simulink model "PQ_VSC_complete_v1"  (R2013b)
settings: Solver=ode45  StartTime=0.0  StopTime=2  MaxStep=0.001  RelTol=1e-3
values from neighbouring files (symbols this model uses):
  Ki = 100    [data_PQsharing.m]
  Ki_PLL = (2*pi*200)^2    (= 1579136.70417)    [data_PQsharing.m]
  Ki_pq = 20    [data_PQsharing.m]
  Kp = 50    [data_PQsharing.m]
  Kp_PLL = sqrt(Ki_PLL)*0.2    [data_PQsharing.m]
  Kp_pq = 0.1    [data_PQsharing.m]
  L = L1    (= 0.04)    [data_PQsharing.m]
  R = 1    [data_PQsharing.m]
  w0 = 377    [data_PQsharing.m]
settings Model: Creator=linglingfan  LastModifiedBy=linglingfan

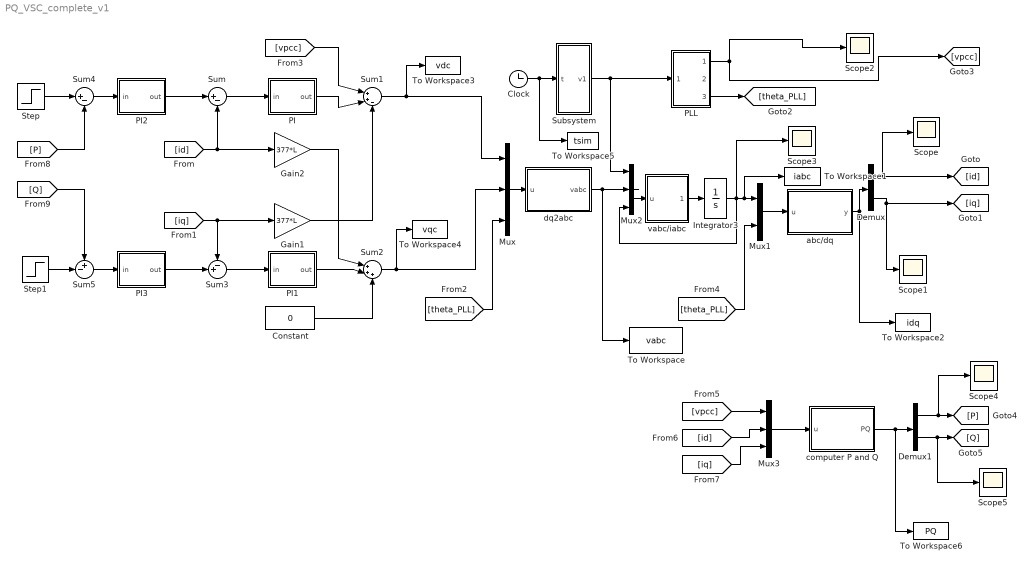
== system PQ_VSC_complete_v1 ==
  Clock : Clock
  Constant : Constant  Value=0
  Demux : Demux  Outputs=2
  Demux1 : Demux  Outputs=2
  Gain1 : Gain  Gain=377*L
  Gain2 : Gain  Gain=377*L
  Integrator3 : Integrator  InitialCondition=zeros(3,1)
  Mux : Mux  Inputs=3
  Mux1 : Mux  Inputs=2
  Mux2 : Mux  Inputs=3
  Mux3 : Mux  Inputs=3
  PI : Subsystem
  PI1 : Subsystem
  PI2 : Subsystem
  PI3 : Subsystem
  PLL : Subsystem
  Scope{,1..5} (6 alike) : Scope
      Scope2 settings: SaveName=ScopeData2
      Scope3 settings: SaveName=ScopeData3
      Scope4 settings: YMin=-6  YMax=7  SaveName=ScopeData4
      Scope5 settings: SaveName=ScopeData5
  Step : Step  Time=0.25  After=0.1  SampleTime=0
  Step1 : Step  After=0.1  SampleTime=0
  Subsystem : Subsystem
  Sum : Sum  Inputs=|+-
  Sum1 : Sum  Inputs=|++-
  Sum2 : Sum  Inputs=|+++
  Sum3 : Sum  Inputs=-+|
  Sum4 : Sum  Inputs=|+-
  Sum5 : Sum  Inputs=+-|
  To Workspace : ToWorkspace  VariableName=vabc  SampleTime=-1
  To Workspace1 : ToWorkspace  VariableName=iabc  SampleTime=-1
  To Workspace2 : ToWorkspace  VariableName=idq  SampleTime=-1
  To Workspace3 : ToWorkspace  VariableName=vdc  SampleTime=-1
  To Workspace4 : ToWorkspace  VariableName=vqc  SampleTime=-1
  To Workspace5 : ToWorkspace  VariableName=tsim  SampleTime=-1
  To Workspace6 : ToWorkspace  VariableName=PQ  SampleTime=-1
  abc/dq : MATLAB Function  TreatAsAtomicUnit=on
  computer P and Q : MATLAB Function  TreatAsAtomicUnit=on
  dq2abc : MATLAB Function  TreatAsAtomicUnit=on
  vabc/iabc : MATLAB Function  TreatAsAtomicUnit=on
  wires:
  Sum/1 -> PI/1(in)
  Mux/1 -> dq2abc/1(u)
  vabc/iabc/1(d_iabc) -> Integrator3/1
  Mux1/1 -> abc/dq/1(u)
  Demux/1 -> Scope/1, [id]
  Demux/2 -> Scope1/1, [iq]
  [id] -> Gain2/1, Sum/2
  [iq] -> Sum3/1, Gain1/1
  Gain2/1 -> Sum2/1
  PI1/1(out) -> Sum2/2
  Constant/1 -> Sum2/3
  [vpcc] -> Sum1/1
  PI/1(out) -> Sum1/2
  Gain1/1 -> Sum1/3
  Sum3/1 -> PI1/1(in)
  PI3/1(out) -> Sum3/2
  PI2/1(out) -> Sum/1
  Sum2/1 -> To Workspace4/1, Mux/2
  Sum1/1 -> To Workspace3/1, Mux/1
  Clock/1 -> To Workspace5/1, Subsystem/1(t)
  Mux2/1 -> vabc/iabc/1(u)
  Subsystem/1(v1) -> PLL/1(abc), Mux2/1
  Integrator3/1 -> Scope3/1, To Workspace1/1, Mux1/1, Mux2/3
  PLL/3(ang) -> [theta_PLL]
  [theta_PLL] -> Mux/3
  dq2abc/1(vabc) -> To Workspace/1, Mux2/2
  PLL/1(mag) -> Scope2/1, [vpcc]
  [theta_PLL] -> Mux1/2
  abc/dq/1(y) -> Demux/1, To Workspace2/1
  [vpcc] -> Mux3/1
  [id] -> Mux3/2
  [iq] -> Mux3/3
  Mux3/1 -> computer P and Q/1(u)
  computer P and Q/1(PQ) -> To Workspace6/1, Demux1/1
  Demux1/1 -> Scope4/1, [P]
  Demux1/2 -> Scope5/1, [Q]
  Sum4/1 -> PI2/1(in)
  Sum5/1 -> PI3/1(in)
  [P] -> Sum4/2
  [Q] -> Sum5/1
  Step/1 -> Sum4/1
  Step1/1 -> Sum5/2

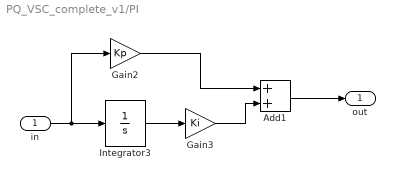
== system PQ_VSC_complete_v1/PI ==
  in : Inport
  Add1 : Sum
  Gain2 : Gain  Gain=Kp
  Gain3 : Gain  Gain=Ki
  Integrator3 : Integrator
  out : Outport
  wires:
  Add1/1 -> out/1
  in/1 -> Gain2/1, Integrator3/1
  Gain3/1 -> Add1/2
  Gain2/1 -> Add1/1
  Integrator3/1 -> Gain3/1

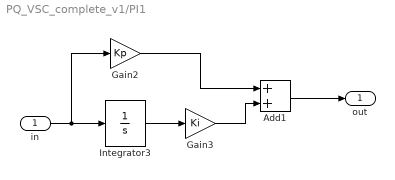
== system PQ_VSC_complete_v1/PI1 ==
  in : Inport
  Add1 : Sum
  Gain2 : Gain  Gain=Kp
  Gain3 : Gain  Gain=Ki
  Integrator3 : Integrator
  out : Outport
  wires:
  Add1/1 -> out/1
  in/1 -> Gain2/1, Integrator3/1
  Gain3/1 -> Add1/2
  Gain2/1 -> Add1/1
  Integrator3/1 -> Gain3/1

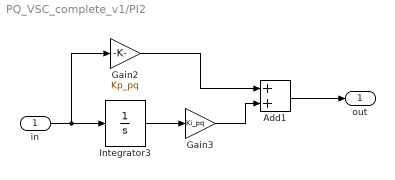
== system PQ_VSC_complete_v1/PI2 ==
  in : Inport
  Add1 : Sum
  Gain2 : Gain  Gain=Kp_pq
  Gain3 : Gain  Gain=Ki_pq
  Integrator3 : Integrator
  out : Outport
  wires:
  Add1/1 -> out/1
  in/1 -> Gain2/1, Integrator3/1
  Gain3/1 -> Add1/2
  Gain2/1 -> Add1/1
  Integrator3/1 -> Gain3/1

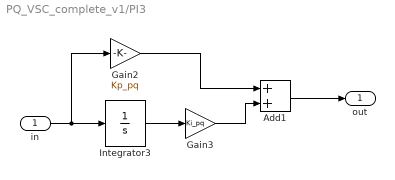
== system PQ_VSC_complete_v1/PI3 ==
  in : Inport
  Add1 : Sum
  Gain2 : Gain  Gain=Kp_pq
  Gain3 : Gain  Gain=Ki_pq
  Integrator3 : Integrator
  out : Outport
  wires:
  Add1/1 -> out/1
  in/1 -> Gain2/1, Integrator3/1
  Gain3/1 -> Add1/2
  Gain2/1 -> Add1/1
  Integrator3/1 -> Gain3/1

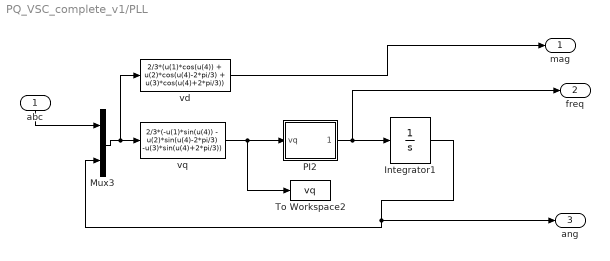
== system PQ_VSC_complete_v1/PLL ==
  abc : Inport
  Integrator1 : Integrator
  Mux3 : Mux  Inputs=2
  PI2 : Subsystem
  To Workspace2 : ToWorkspace  VariableName=vq  SampleTime=-1
  vd : Fcn  Expr=2/3*(u(1)*cos(u(4)) + u(2)*cos(u(4)-2*pi/3) + u(3)*cos(u(4)+2*pi/3))
  vq : Fcn  Expr=2/3*(-u(1)*sin(u(4)) - u(2)*sin(u(4)-2*pi/3) -u(3)*sin(u(4)+2*pi/3))
  mag : Outport
  freq : Outport  Port=2
  ang : Outport  Port=3
  wires:
  Mux3/1 -> vd/1, vq/1
  PI2/1(omega) -> freq/1, Integrator1/1
  abc/1 -> Mux3/1
  vq/1 -> To Workspace2/1, PI2/1(vq)
  vd/1 -> mag/1
  Integrator1/1 -> ang/1, Mux3/2

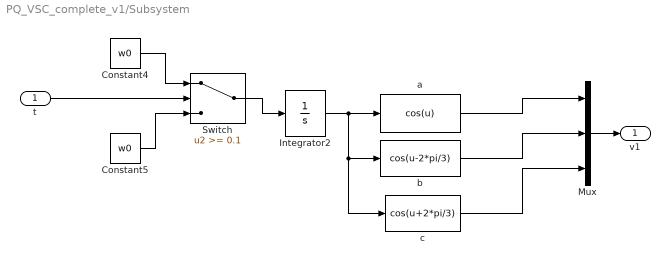
== system PQ_VSC_complete_v1/Subsystem ==
  t : Inport
  Constant4 : Constant  Value=w0
  Constant5 : Constant  Value=w0
  Integrator2 : Integrator
  Mux : Mux  Inputs=3
  Switch : Switch  Threshold=0.1
  a : Fcn  Expr=cos(u)
  b : Fcn  Expr=cos(u-2*pi/3)
  c : Fcn  Expr=cos(u+2*pi/3)
  v1 : Outport
  wires:
  a/1 -> Mux/1
  c/1 -> Mux/3
  Integrator2/1 -> c/1, b/1, a/1
  b/1 -> Mux/2
  t/1 -> Switch/2
  Constant4/1 -> Switch/1
  Switch/1 -> Integrator2/1
  Constant5/1 -> Switch/3
  Mux/1 -> v1/1

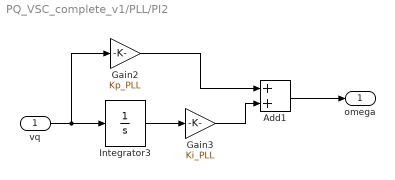
== system PQ_VSC_complete_v1/PLL/PI2 ==
  vq : Inport
  Add1 : Sum
  Gain2 : Gain  Gain=Kp_PLL
  Gain3 : Gain  Gain=Ki_PLL
  Integrator3 : Integrator
  omega : Outport
  wires:
  Add1/1 -> omega/1
  vq/1 -> Gain2/1, Integrator3/1
  Gain3/1 -> Add1/2
  Gain2/1 -> Add1/1
  Integrator3/1 -> Gain3/1

== matlab function PQ_VSC_complete_v1/vabc//iabc ==
  data: u input; d_iabc output; R parameter; L parameter
function d_iabc = fcn_vabc2iabc(u, R, L)
%#codegen
v1a = u(1); 
v1b = u(2); 
v1c = u(3); 
va = u(4); 
vb = u(5); 
vc = u(6); 
ia = u(7); ib = u(8); ic = u(9);
d_iabc = 1/L*[va- v1a - R*ia; vb-v1b-R*ib; vc-v1c-R*ic];

== matlab function PQ_VSC_complete_v1/dq2abc ==
  data: u input; vabc output
function vabc = fcn(u)
%#codegen
dq = u(1:2);
theta = u(3);
A =[cos(theta), -sin(theta); 
    cos(theta-2*pi/3), -sin(theta-2*pi/3); 
    cos(theta+2*pi/3), -sin(theta+2*pi/3)];

vabc = A*dq;

== matlab function PQ_VSC_complete_v1/abc//dq ==
  data: u input; y output
function y = fcn_abc2dq(u)
%#codegen

abc = u(1:3);
theta = u(4);
A =2/3*[cos(theta), cos(theta-2*pi/3),  cos(theta+2*pi/3); 
-sin(theta), -sin(theta-2*pi/3),  -sin(theta+2*pi/3)];

y = A*abc;

== matlab function PQ_VSC_complete_v1/computer P and Q ==
  data: u input; PQ output
function PQ = fcn(u)
%#codegen
% use per unit-value instead of per unit value. 
% real value: P = 1.5*v*id. 
% here we assume v_b = 1, id_base =1; then P_pu = v*id. 
v = u(1); id = u(2); iq = u(3); 
P = v*id;
Q = -v*iq; 
PQ =[P; Q];
